simulink model "citt_generated_model"  (R2026b)
settings: Solver=ode23t  StopTime=t_stop  MaxStep=max_step
model workspace (MAT data in the model file):
  A_ol = 20000
  A_ol_values = [1000 3000 10000 30000 100000]
  C_m = 5e-10
  E_leak = -0.065
  I_leak = 3.25e-09
  I_limit = 5e-09
  I_membrane_nonlinear_max = 5e-10
  I_nl = 0
  K_ctrl = 1
  N_bits = 12
  R_e = 2000000
  R_e_values = [200000 500000 1000000 2000000 5000000]
  R_m = 20000000
  R_series_output = 100000
  T_s = 0.0002
  V_adc_ref = 0.4
  V_c = -0.02
  V_c_initial = -0.065
  V_cmd_final = -0.02
  V_cmd_initial = -0.065
  V_nonlinear_slope = 0.006
  V_nonlinear_threshold = -0.04
  V_rail_minus = -1
  V_rail_plus = 1
  V_rest = -0.065
  adc_bits = 12
  adc_input_range = [-0.2 0.2]
  adc_lsb = 9.765625e-05
  amplifier_bandwidth_hz = 2000
  command_step_time = 0.005
  digital_settled_hold_time = 0.002
  digital_settled_threshold = 0.001
  fs = 5000
  input_noise_rms = 0.0001
  input_offset = 0
  max_step = 1e-05
  output_current_limit = 5e-09
  output_rails = [-1 1]
  output_resistance = 50
  parameter_set_label = "educational scaled benchmark parameters"
  parameter_set_warning = "Not a clinically validated axon model."
  saturation_current_threshold = 4.8e-09
  saturation_voltage_threshold = 0.95
  t_step = 0.005
  t_stop = 0.06
libraries: fl_lib x15, nesl_utility x7, ee_lib x4, simulink x3
settings Model: Creator=Raalm  LastModifiedBy=Raalm
settings SimscapeCC: SimscapeLogType=all  SimscapeNominalValues="[{\"value\":\"1\",\"unit\":\"A\"},{\"value\":\"1\",\"unit\":\"bar\"},{\"value\":\"1\",\"unit\":\"cm^2\"},{\"value\":\"1\",\"unit\":\"cm^3/s\"},{\"value\":\"1\",\"unit\":\"kJ/kg\"},{\"value\":\"1\",\"unit\":\"kW\"},{\"value\":\"1\",\"unit\":\"l\"},{\"value\":\"1\",\"unit\":\"N\"},{\"value\":\"1\",\"unit\":\"N*m\"},{\"value\":\"1\",\"unit\":\"V\"},{\"value\":\"0.001\",\"unit\":\"Wb\"}]"  SimscapeUseEnergyAccounting=off

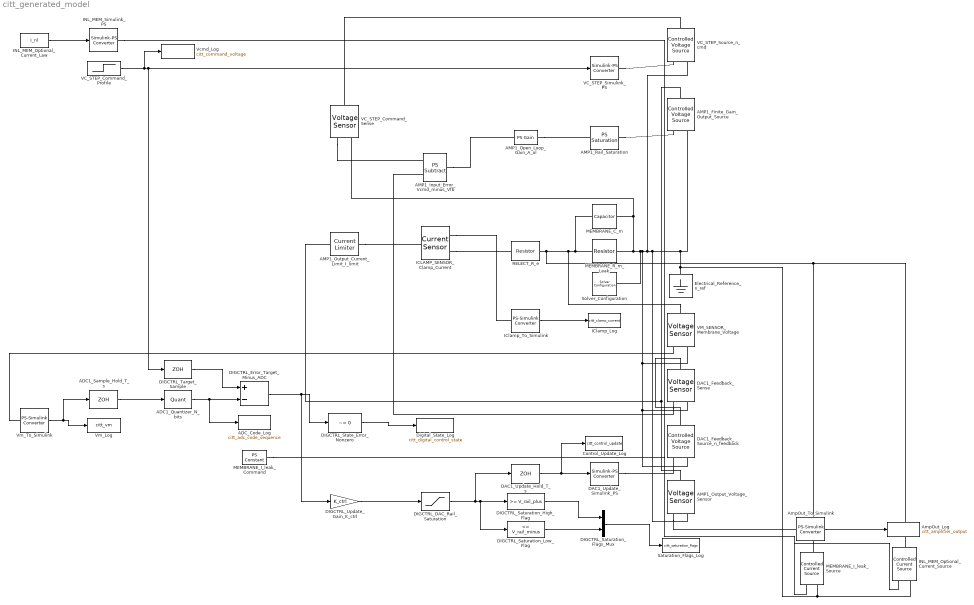
== system citt_generated_model ==
  ADC1_Quantizer_N_bits : Quantizer  QuantizationInterval=V_adc_ref/(2^N_bits - 1)  SampleTime=T_s
  ADC1_Sample_Hold_T_s : ZeroOrderHold  SampleTime=T_s
  ADC_Code_Log : ToWorkspace  VariableName=citt_adc_code_sequence  SaveFormat=Timeseries  SampleTime=-1
  AMP1_Finite_Gain_Output_Source : fl_lib/Electrical/Electrical Sources/Controlled Voltage Source
  AMP1_Input_Error_Vcmd_minus_Vfb : fl_lib/Physical Signals/Functions/PS Subtract
  AMP1_Open_Loop_Gain_A_ol : fl_lib/Physical Signals/Functions/PS Gain  gain=A_ol
  AMP1_Output_Current_Limit_I_limit : ee_lib/Semiconductors & Converters/Current Limiter  limType=ee.enum.semiconductors.currLimType.constLim  iLim=I_limit A  iLimReverse=I_limit A  vLim=0.1 V  gLim=1e-10 1/Ohm  thermal_mass=100 J/K  temperature_specify=off  temperature_priority=High  temperature=298.15 K  temperature_nominal_specify=off  temperature_nominal_value=1  temperature_nominal_unit=K
  AMP1_Output_Voltage_Sensor : fl_lib/Electrical/Electrical Sensors/Voltage Sensor
  AMP1_Rail_Saturation : fl_lib/Physical Signals/Nonlinear Operators/PS Saturation  upper_limit=V_rail_plus V  lower_limit=V_rail_minus V  ZeroCross=true
  AmpOut_Log : ToWorkspace  VariableName=citt_amplifier_output  SaveFormat=Timeseries  SampleTime=-1
  AmpOut_To_Simulink : nesl_utility/PS-Simulink Converter  PhysicalDomain=network_engine_domain  SubClassName=ps_output  LeftPortType=input  RightPortType=output  PseudoPeriodic=off  Frequencies=[]  VectorFormat=inherit  Unit=V  AffineConversion=off
  Control_Update_Log : ToWorkspace  VariableName=citt_control_update  SaveFormat=Timeseries  SampleTime=-1
  DAC1_Feedback_Sense : fl_lib/Electrical/Electrical Sensors/Voltage Sensor
  DAC1_Feedback_Source_n_feedback : fl_lib/Electrical/Electrical Sources/Controlled Voltage Source
  DAC1_Update_Hold_T_s : ZeroOrderHold  SampleTime=T_s
  DAC1_Update_Simulink_PS : nesl_utility/Simulink-PS Converter  PhysicalDomain=network_engine_domain  SubClassName=ps_input  LeftPortType=input  RightPortType=output  PseudoPeriodic=off  Frequencies=[]  NoiseDistribution=none  NoiseParameters=[]  Unit=V  AffineConversion=off  FilteringAndDerivatives=provide  SimscapeFilterOrder=1  InputFilterTimeConstant=0.001  UdotUserProvided=0
  DIGCTRL_DAC_Rail_Saturation : Saturate  UpperLimit=V_rail_plus  LowerLimit=V_rail_minus
  DIGCTRL_Error_Target_Minus_ADC : Sum  Inputs=+-
  DIGCTRL_Saturation_Flags_Mux : Mux  Inputs=2
  DIGCTRL_Saturation_High_Flag : simulink/Logic and Bit Operations/Compare To Constant  relop=>=  const=V_rail_plus  OutDataTypeStr=boolean
  DIGCTRL_Saturation_Low_Flag : simulink/Logic and Bit Operations/Compare To Constant  relop=<=  const=V_rail_minus  OutDataTypeStr=boolean
  DIGCTRL_State_Error_Nonzero : simulink/Logic and Bit Operations/Compare To Constant  relop=~=  const=0  OutDataTypeStr=boolean
  DIGCTRL_Target_Sample : ZeroOrderHold  SampleTime=T_s
  DIGCTRL_Update_Gain_K_ctrl : Gain  Gain=K_ctrl
  Digital_State_Log : ToWorkspace  VariableName=citt_digital_control_state  SaveFormat=Timeseries  SampleTime=-1
  Electrical_Reference_n_ref : fl_lib/Electrical/Electrical Elements/Electrical Reference
  ICLAMP_SENSOR_Clamp_Current : fl_lib/Electrical/Electrical Sensors/Current Sensor
  IClamp_Log : ToWorkspace  VariableName=citt_clamp_current  SaveFormat=Timeseries  SampleTime=-1
  IClamp_To_Simulink : nesl_utility/PS-Simulink Converter  PhysicalDomain=network_engine_domain  SubClassName=ps_output  LeftPortType=input  RightPortType=output  PseudoPeriodic=off  Frequencies=[]  VectorFormat=inherit  Unit=A  AffineConversion=off
  INL_MEM_Optional_Current_Law : Constant  Value=I_nl
  INL_MEM_Optional_Current_Source : fl_lib/Electrical/Electrical Sources/Controlled Current Source
  INL_MEM_Simulink_PS : nesl_utility/Simulink-PS Converter  PhysicalDomain=network_engine_domain  SubClassName=ps_input  LeftPortType=input  RightPortType=output  PseudoPeriodic=off  Frequencies=[]  NoiseDistribution=none  NoiseParameters=[]  Unit=A  AffineConversion=off  FilteringAndDerivatives=provide  SimscapeFilterOrder=1  InputFilterTimeConstant=0.001  UdotUserProvided=0
  MEMBRANE_C_m : ee_lib/Passive/Capacitor  cap_option=ee.enum.passive.capacitor.capOption.const  c=C_m F  Cvec=[1e-05, 1e-06] F  Vvec=[0, 10] V  CV_table_symmetry=ee.enum.passive.capacitor.tableSymmetry.yes  f_vec=[1, 10] kHz  DFext_vec=[.8, 1.2]  enable_C_tol=ee.enum.toleranceApplication.none  averaging_period=0 s  C_tol=5  tol_distribution=ee.enum.toleranceDistribution.uniform  nSigma=4  r=0 Ohm  g=0 1/Ohm  enable_operating_limits=ee.enum.enable.no  operating_limit_action=ee.enum.passive.reportOpLim.warn  max_working_voltage_range=[-25, 25] V  power_rating=1 W  maxTemperature=85 degC  thermalEnable=false  thermalMass=1 J/K  i_specify=off  i_priority=None  i=0 A  i_nominal_specify=off  i_nominal_value=1  i_nominal_unit=A  v_specify=off  v_priority=High  v=V_rest V  v_nominal_specify=off  v_nominal_value=1  v_nominal_unit=V  vc_specify=off  vc_priority=High  vc=V_rest V  vc_nominal_specify=off  vc_nominal_value=1  vc_nominal_unit=V  T_specify=off  T_priority=None  T=298.15 K  T_nominal_specify=off  T_nominal_value=1  T_nominal_unit=K
  MEMBRANE_I_leak_Command : fl_lib/Physical Signals/Sources/PS Constant  constant=I_leak A
  MEMBRANE_I_leak_Source : fl_lib/Electrical/Electrical Sources/Controlled Current Source
  MEMBRANE_R_m_Leak : ee_lib/Passive/Resistor  R=R_m Ohm  enable_R_tol=ee.enum.toleranceApplication.none  R_tol=5  tol_distribution=ee.enum.toleranceDistribution.uniform  nSigma=4  enable_operating_limits=ee.enum.enable.no  operating_limit_action=ee.enum.passive.reportOpLim.warn  power_rating=1 W  max_working_voltage=100 V  noise_mode=ee.enum.sources.noise.Disabled  Tdevice=25 degC  sample_time=1e-3 s  repeatability=ee.enum.ic.repeatability.notRepeatable  user_seed=0  auto_seed=1019125215  power_derating_T1=70 degC  power_derating_T2=155 degC  operating_temperature_range_vec=[-50, 150] degC  alpha=3.93e-3 1/K  Tmeas=25 degC  thermal_mass=100 J/K  temperature_specify=off  temperature_priority=High  temperature=298.15 K  temperature_nominal_specify=off  temperature_nominal_value=1  temperature_nominal_unit=K
  RELECT_R_e : ee_lib/Passive/Resistor  R=R_e Ohm  enable_R_tol=ee.enum.toleranceApplication.none  R_tol=5  tol_distribution=ee.enum.toleranceDistribution.uniform  nSigma=4  enable_operating_limits=ee.enum.enable.no  operating_limit_action=ee.enum.passive.reportOpLim.warn  power_rating=1 W  max_working_voltage=100 V  noise_mode=ee.enum.sources.noise.Disabled  Tdevice=25 degC  sample_time=1e-3 s  repeatability=ee.enum.ic.repeatability.notRepeatable  user_seed=0  auto_seed=2484746217  power_derating_T1=70 degC  power_derating_T2=155 degC  operating_temperature_range_vec=[-50, 150] degC  alpha=3.93e-3 1/K  Tmeas=25 degC  thermal_mass=100 J/K  temperature_specify=off  temperature_priority=High  temperature=298.15 K  temperature_nominal_specify=off  temperature_nominal_value=1  temperature_nominal_unit=K
  Saturation_Flags_Log : ToWorkspace  VariableName=citt_saturation_flags  SaveFormat=Timeseries  SampleTime=-1
  Solver_Configuration : nesl_utility/Solver Configuration  PhysicalDomain=network_engine_domain  SubClassName=solver  LeftPortType=input  RightPortType=generic  Tones=[]  Harmonics=[]  SimulateNoise=off  Profile=off  UseLocalSampling=off  EnableSwitchedLinearOptims=on  FrequencyDomain=off  UseCCode=off  RelTol=0.001  AbsTol=0.001  MinStep=1e-09  ToWorkspace=off  RevertToSquareIcSolve=off  NumHomotopyIterations=100  PhasorMode=off  PhasorModeNumHarmonics=1  ConsistencySolver=NEWTON_XTOL_AFTER_FTOL  CanonicalOrdering=CANONICAL  OptimizeIntermediates=OPTIMIZED  MulticoreSolverChoice=BACKWARD_EULER  IndexReductionMethod=DerivativeReplacement  DoDC=off  ResidualTolerance=1e-09  ConsistencyTolSource=GLOBAL  ConsistencyAbsTol=0.001  ConsistencyRelTol=0.001  ConsistencyTolFactor=0.001  UseLocalSolver=off  LocalSolverChoice=NE_BACKWARD_EULER_ADVANCER  ResolveIndetEquations=on  FunctionEvalNumThread=1  LocalSolverSampleTime=0.001  DoFixedCost=off  MaxNonlinIter=3  MaxModeIter=2  ComputeImpulses=off  ImpulseIterations=2  LinearAlgebra=auto  LinearAlgebraNumThread=0  EquationFormulation=NE_TIME_EF  DelaysMemoryBudget=1024  AutomaticFiltering=on  FilteringTimeConstant=0.001  PartitionStorageMethod=AS_NEEDED  PartitionMemoryBudget=1024  PartitionMethod=BALANCED  MultibodyUseLocalSolver=off  MultibodyLocalSolverChoice=ODE1  MultibodyLocalSolverSampleTime=0.001
  VC_STEP_Command_Profile : Step  Time=t_step  InitialValue=V_c_initial  FinalValue=V_c  SampleTime=0
  VC_STEP_Command_Sense : fl_lib/Electrical/Electrical Sensors/Voltage Sensor
  VC_STEP_Simulink_PS : nesl_utility/Simulink-PS Converter  PhysicalDomain=network_engine_domain  SubClassName=ps_input  LeftPortType=input  RightPortType=output  PseudoPeriodic=off  Frequencies=[]  NoiseDistribution=none  NoiseParameters=[]  Unit=V  AffineConversion=off  FilteringAndDerivatives=provide  SimscapeFilterOrder=1  InputFilterTimeConstant=0.001  UdotUserProvided=0
  VC_STEP_Source_n_cmd : fl_lib/Electrical/Electrical Sources/Controlled Voltage Source
  VM_SENSOR_Membrane_Voltage : fl_lib/Electrical/Electrical Sensors/Voltage Sensor
  Vcmd_Log : ToWorkspace  VariableName=citt_command_voltage  SaveFormat=Timeseries  SampleTime=-1
  Vm_Log : ToWorkspace  VariableName=citt_vm  SaveFormat=Timeseries  SampleTime=-1
  Vm_To_Simulink : nesl_utility/PS-Simulink Converter  PhysicalDomain=network_engine_domain  SubClassName=ps_output  LeftPortType=input  RightPortType=output  PseudoPeriodic=off  Frequencies=[]  VectorFormat=inherit  Unit=V  AffineConversion=off
  wires:
  DIGCTRL_Saturation_Flags_Mux/1 -> Saturation_Flags_Log/1
  DIGCTRL_Saturation_Low_Flag/1 -> DIGCTRL_Saturation_Flags_Mux/2
  DIGCTRL_Saturation_High_Flag/1 -> DIGCTRL_Saturation_Flags_Mux/1
  DIGCTRL_State_Error_Nonzero/1 -> Digital_State_Log/1
  DAC1_Update_Hold_T_s/1 -> DAC1_Update_Simulink_PS/1, Control_Update_Log/1
  DIGCTRL_DAC_Rail_Saturation/1 -> DIGCTRL_Saturation_High_Flag/1, DIGCTRL_Saturation_Low_Flag/1, DAC1_Update_Hold_T_s/1
  DIGCTRL_Update_Gain_K_ctrl/1 -> DIGCTRL_DAC_Rail_Saturation/1
  DIGCTRL_Error_Target_Minus_ADC/1 -> DIGCTRL_Update_Gain_K_ctrl/1, DIGCTRL_State_Error_Nonzero/1
  DIGCTRL_Target_Sample/1 -> DIGCTRL_Error_Target_Minus_ADC/1
  ADC1_Quantizer_N_bits/1 -> DIGCTRL_Error_Target_Minus_ADC/2, ADC_Code_Log/1
  ADC1_Sample_Hold_T_s/1 -> ADC1_Quantizer_N_bits/1
  INL_MEM_Optional_Current_Law/1 -> INL_MEM_Simulink_PS/1
  AmpOut_To_Simulink/1 -> AmpOut_Log/1
  IClamp_To_Simulink/1 -> IClamp_Log/1
  Vm_To_Simulink/1 -> Vm_Log/1, ADC1_Sample_Hold_T_s/1
  VC_STEP_Command_Profile/1 -> VC_STEP_Simulink_PS/1, DIGCTRL_Target_Sample/1, Vcmd_Log/1
  connections:
  DAC1_Feedback_Source_n_feedback/LConn1 -- DAC1_Feedback_Sense/LConn1
  DAC1_Update_Simulink_PS/RConn1 -- DAC1_Feedback_Source_n_feedback/RConn1
  AMP1_Output_Voltage_Sensor/RConn1 -- AmpOut_To_Simulink/LConn1
  ICLAMP_SENSOR_Clamp_Current/RConn1 -- IClamp_To_Simulink/LConn1
  VM_SENSOR_Membrane_Voltage/RConn1 -- Vm_To_Simulink/LConn1
  VM_SENSOR_Membrane_Voltage/LConn1 -- MEMBRANE_R_m_Leak/LConn1 -- MEMBRANE_C_m/LConn1 -- MEMBRANE_I_leak_Source/LConn1 -- INL_MEM_Optional_Current_Source/LConn1 -- RELECT_R_e/RConn1
  ICLAMP_SENSOR_Clamp_Current/RConn2 -- RELECT_R_e/LConn1
  AMP1_Output_Current_Limit_I_limit/RConn1 -- ICLAMP_SENSOR_Clamp_Current/LConn1
  AMP1_Finite_Gain_Output_Source/LConn1 -- AMP1_Output_Voltage_Sensor/LConn1 -- AMP1_Output_Current_Limit_I_limit/LConn1
  AMP1_Rail_Saturation/RConn1 -- AMP1_Finite_Gain_Output_Source/RConn1
  AMP1_Open_Loop_Gain_A_ol/RConn1 -- AMP1_Rail_Saturation/LConn1
  AMP1_Input_Error_Vcmd_minus_Vfb/RConn1 -- AMP1_Open_Loop_Gain_A_ol/LConn1
  DAC1_Feedback_Sense/RConn1 -- AMP1_Input_Error_Vcmd_minus_Vfb/LConn2
  VC_STEP_Command_Sense/RConn1 -- AMP1_Input_Error_Vcmd_minus_Vfb/LConn1
  VC_STEP_Source_n_cmd/LConn1 -- VC_STEP_Command_Sense/LConn1
  VC_STEP_Simulink_PS/RConn1 -- VC_STEP_Source_n_cmd/RConn1
  Solver_Configuration/RConn1 -- DAC1_Feedback_Source_n_feedback/RConn2 -- DAC1_Feedback_Sense/RConn2 -- VM_SENSOR_Membrane_Voltage/RConn2 -- MEMBRANE_I_leak_Source/RConn2 -- INL_MEM_Optional_Current_Source/RConn2 -- Electrical_Reference_n_ref/LConn1 -- AMP1_Finite_Gain_Output_Source/RConn2 -- AMP1_Output_Voltage_Sensor/RConn2 -- VC_STEP_Source_n_cmd/RConn2 -- VC_STEP_Command_Sense/RConn2 -- MEMBRANE_C_m/RConn1 -- MEMBRANE_R_m_Leak/RConn1
  MEMBRANE_I_leak_Command/RConn1 -- MEMBRANE_I_leak_Source/RConn1
  INL_MEM_Simulink_PS/RConn1 -- INL_MEM_Optional_Current_Source/RConn1
